simulink model "simulink_daq_module"  (Simulink 7.5)
settings: Solver=FixedStepDiscrete  SolverMode=SingleTasking  StartTime=0.0  StopTime=inf  FixedStep=1/500  RelTol=1e-3
settings Model: Creator=breidi  LastModifiedBy=breidi
settings SolverCC: InsertRTBMode=Never (minimum delay)
settings DataIOCC: LimitDataPoints=off  SaveOutput=off  SignalLogging=off  SaveTime=off
settings OptimizationCC: InlineParams=on  InlineInvariantSignals=on  EnhancedBackFolding=on  EfficientFloat2IntCast=on  SimCompilerOptimization=On
settings DebuggingCC: StrictBusMsg=Warning

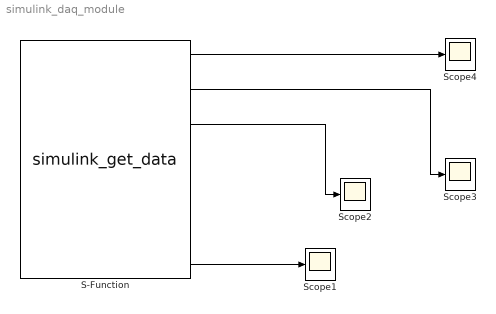
== system simulink_daq_module ==
  S-Function : S-Function  Priority=1  FunctionName=simulink_get_data  Parameters=master_info, sig_info, ch_info, server_info  EnableBusSupport=off  mask{ip='127.0.0.1', port=9000, proto='udp'}
      mask prompts: ip "Server IP"; proto "Protocol"
      mask init:
      | global master_info;
      | global sig_info;
      | global ch_info;
      | global fs;
      | 
      | fs = 0;
      | bs = 0;
      | 
      | [master_info sig_info ch_info server_info_tmp] = mex_get_config(ip, port, proto);
      | server_info{1} = proto;
      | server_info{2} = ip;
      | server_info{3} = server_info_tmp;
      | 
      | disp(' ');
      | disp(' ----------------------------------------------------------------------------------------------------- ');
      | disp(' ');
      | disp(' ***** NOTICE: Initialization done in "Net Signal Client" -> Edit Mask -> Initialization! ***** ');
      | 
      | disp(' ');
      | disp('SignalServer Information (protocol, server-IP, server-port):');
      | disp(server_info);
      | 
      | disp(' ');
      | disp('Master Sampling Rate and Blocksize:');
      | disp(master_info);
      | disp('Signal Types Info:  (Flag, Type, BS, NrCh, Fs)');
      | disp(sig_info);
      | disp('Channel Info:  (Name, Type)');
      | disp(ch_info);
      | disp(' ');
      | 
      | fs = master_info(1);
      | bs = master_info(2);
      | 
      | % for n = 1:size(sig_info,1)
      | % %   port_label('output', 1, num2str(cell2mat(sig_info(n,2))) );
      | % end
      | % port_label('input', 1, 'a');
      | % num2str(cell2mat(sig_info(n,2)))
      | 
      | set_param(gcs, 'SolverName', 'FixedStepDiscrete');
      | set_param(gcs, 'FixedStep', [ num2str(1) '/' num2str(fs)])
      | % set_param(gcs, 'SolverMode', 'Auto');
      | % set_param(gcs, 'FixedStep', '1');
      mask Display:
      | disp('TOBI Signal\nClient')
      | port_label('output', 1, num2str(cell2mat(sig_info(1,2))) );
      | 
      | port_label('output', size(sig_info,1)+1, 'events' );
      | port_label('output', size(sig_info,1)+2, 'sample nr' );
      | port_label('output', size(sig_info,1)+3, 'timestamp' );
      | port_label('output', size(sig_info,1)+4, 'sys/sim time' );
  Scope{1..4} (4 alike) : Scope
      Scope1 settings: TimeRange=1  YMin=-1500  YMax=6500
      Scope2 settings: TimeRange=1  YMin=-22500  YMax=30000  SaveName=ScopeData2
      Scope3 settings: TimeRange=1  YMin=-1500  YMax=6500
      Scope4 settings: TimeRange=1  YMin=-1500  YMax=6500  SaveName=ScopeData3
  wires:
  S-Function/3 -> Scope2/1
  S-Function/7 -> Scope1/1
  S-Function/2 -> Scope3/1
  S-Function/1 -> Scope4/1
